simulink library "vehicle_model"  (R2018b)
settings: Solver=ode45  StartTime=0.0  StopTime=10.0  RelTol=1e-3  EnableMultiTasking=on
undefined symbols (not defined in the file): DiscIntNeverNeededParam, par_VEH, select_To_Wks_akt, stepsize, v0
libraries: $bdroot x8, pacejka_trans x6, simulink x4, body_chassis_vert x1
(part 1 of 4)
settings Model: Creator=CA-Win7Pro2  LastModifiedBy=ga35gug
settings DataIOCC: LimitDataPoints=on  SaveFormat=Array  SignalLoggingSaveFormat=ModelDataLogs
settings OptimizationCC: LifeSpan=inf
settings DebuggingCC: UnderspecifiedInitializationDetection=Classic  MergeDetectMultiDrivingBlocksExec=none  SolverPrmCheckMsg=warning  MultiTaskDSMMsg=warning  MultiTaskCondExecSysMsg=none  AllowSymbolicDim=off  SFUnexpectedBacktrackingDiag=warning  SFNoUnconditionalDefaultTransitionDiag=warning  SFExecutionAtInitializationDiag=none
settings HardwareCC: ProdBitPerPointer=32  ProdBitPerSizeT=32  ProdBitPerPtrDiffT=32  ProdLargestAtomicFloat=None  ProdIntDivRoundTo=Undefined  ProdEndianess=Unspecified  ProdWordSize=32  ProdHWDeviceType=32-bit Generic
settings ModelReferenceCC: PropagateSignalLabelsOutOfModel=off
settings SFSimCC: SimUseLocalCustomCode=off
settings RTWCC: RTWUseLocalCustomCode=off
settings CodeAppCC: StateflowObjectComments=on
settings GRTTargetCC: TargetLangStandard=C89/C90 (ANSI)  GeneratePreprocessorConditionals=Disable all
settings ConfigComp: CovMetricSettings=dw  CovHtmlReporting=on  CovSaveCumulativeToWorkspaceVar=on  CovSaveSingleToWorkspaceVar=on  CovExternalEMLEnable=off

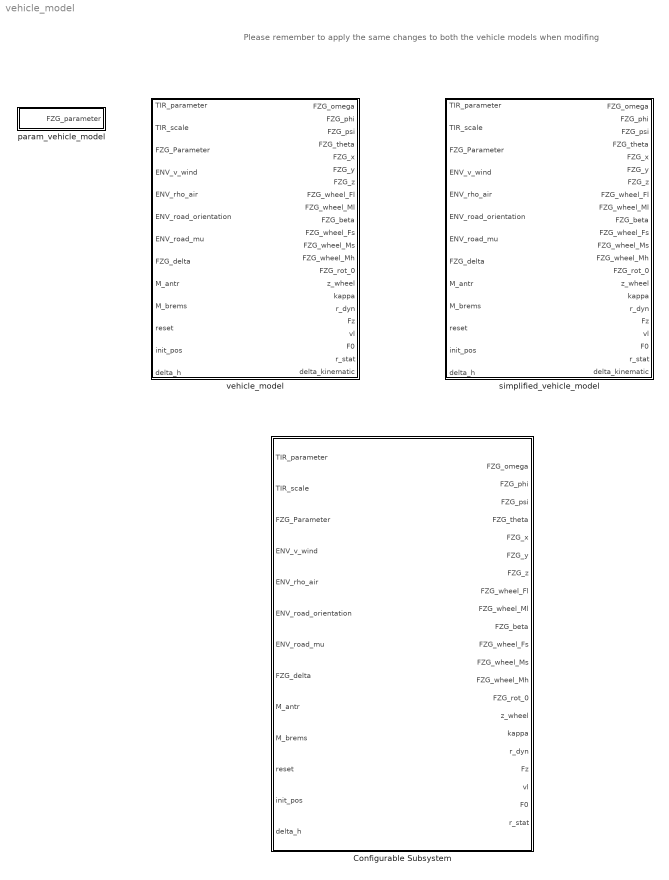
== system vehicle_model ==
  note: Please remember to apply the same changes to both the vehicle models when modifing
  Configurable Subsystem : Subsystem  BlockChoice=vehicle_model
      settings: TemplateBlock=self  MemberBlocks=simplified_vehicle_model,vehicle_model
  param_vehicle_model : Subsystem
  simplified_vehicle_model : Subsystem  TreatAsAtomicUnit=on  SystemSampleTime=stepsize
      settings: MinAlgLoopOccurrences=on
  vehicle_model : Subsystem  TreatAsAtomicUnit=on  SystemSampleTime=stepsize
      settings: MinAlgLoopOccurrences=on

== system vehicle_model/Configurable Subsystem ==
  TIR_parameter : Inport
  TIR_scale : Inport  Port=2
  FZG_Parameter : Inport  Port=3
  ENV_v_wind : Inport  Port=4
  ENV_rho_air : Inport  Port=5
  ENV_road_orientation : Inport  Port=6
  ENV_road_mu : Inport  Port=7
  FZG_delta : Inport  Port=8
  M_antr : Inport  Port=9
  M_brems : Inport  Port=10
  reset : Inport  Port=11
  init_pos : Inport  Port=12
  delta_h : Inport  Port=13
  vehicle_model : $bdroot/vehicle_model  SystemSampleTime=stepsize
  FZG_omega : Outport
  FZG_phi : Outport  Port=2
  FZG_psi : Outport  Port=3
  FZG_theta : Outport  Port=4
  FZG_x : Outport  Port=5
  FZG_y : Outport  Port=6
  FZG_z : Outport  Port=7
  FZG_wheel_Fl : Outport  Port=8
  FZG_wheel_Ml : Outport  Port=9
  FZG_beta : Outport  Port=10
  FZG_wheel_Fs : Outport  Port=11
  FZG_wheel_Ms : Outport  Port=12
  FZG_wheel_Mh : Outport  Port=13
  FZG_rot_0 : Outport  Port=14
  z_wheel : Outport  Port=15
  kappa : Outport  Port=16
  r_dyn : Outport  Port=17
  Fz : Outport  Port=18
  vl : Outport  Port=19
  F0 : Outport  Port=20
  r_stat : Outport  Port=21
  wires:
  TIR_parameter/1 -> vehicle_model/1
  TIR_scale/1 -> vehicle_model/2
  FZG_Parameter/1 -> vehicle_model/3
  ENV_v_wind/1 -> vehicle_model/4
  ENV_rho_air/1 -> vehicle_model/5
  ENV_road_orientation/1 -> vehicle_model/6
  ENV_road_mu/1 -> vehicle_model/7
  FZG_delta/1 -> vehicle_model/8
  M_antr/1 -> vehicle_model/9
  M_brems/1 -> vehicle_model/10
  reset/1 -> vehicle_model/11
  init_pos/1 -> vehicle_model/12
  delta_h/1 -> vehicle_model/13
  vehicle_model/1 -> FZG_omega/1
  vehicle_model/2 -> FZG_phi/1
  vehicle_model/3 -> FZG_psi/1
  vehicle_model/4 -> FZG_theta/1
  vehicle_model/5 -> FZG_x/1
  vehicle_model/6 -> FZG_y/1
  vehicle_model/7 -> FZG_z/1
  vehicle_model/8 -> FZG_wheel_Fl/1
  vehicle_model/9 -> FZG_wheel_Ml/1
  vehicle_model/10 -> FZG_beta/1
  vehicle_model/11 -> FZG_wheel_Fs/1
  vehicle_model/12 -> FZG_wheel_Ms/1
  vehicle_model/13 -> FZG_wheel_Mh/1
  vehicle_model/14 -> FZG_rot_0/1
  vehicle_model/15 -> z_wheel/1
  vehicle_model/16 -> kappa/1
  vehicle_model/17 -> r_dyn/1  "kappa"
  vehicle_model/18 -> Fz/1  "Fz"
  vehicle_model/19 -> vl/1  "vl"
  vehicle_model/20 -> F0/1  "F0"
  vehicle_model/21 -> r_stat/1

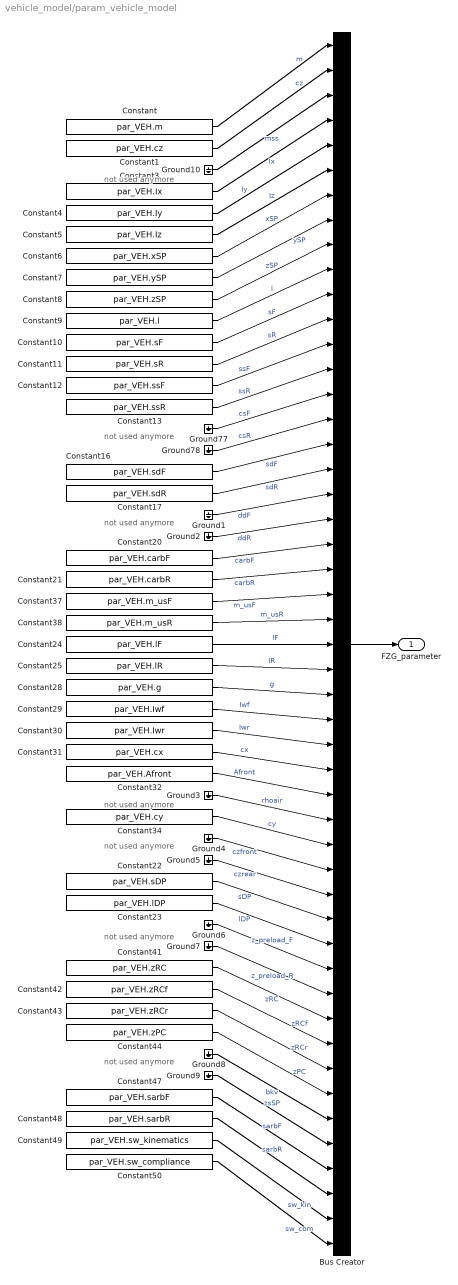
== system vehicle_model/param_vehicle_model ==
  note: not used anymore
  note: not used anymore
  note: not used anymore
  note: not used anymore
  note: not used anymore
  note: not used anymore
  note: not used anymore
  Bus Creator : BusCreator  Inputs=49
  Constant : Constant  Value=par_VEH.m
  Constant1 : Constant  Value=par_VEH.cz
  Constant10 : Constant  Value=par_VEH.sF
  Constant11 : Constant  Value=par_VEH.sR
  Constant12 : Constant  Value=par_VEH.ssF
  Constant13 : Constant  Value=par_VEH.ssR
  Constant16 : Constant  Value=par_VEH.sdF
  Constant17 : Constant  Value=par_VEH.sdR
  Constant20 : Constant  Value=par_VEH.carbF
  Constant21 : Constant  Value=par_VEH.carbR
  Constant22 : Constant  Value=par_VEH.sDP
  Constant23 : Constant  Value=par_VEH.lDP
  Constant24 : Constant  Value=par_VEH.lF
  Constant25 : Constant  Value=par_VEH.lR
  Constant28 : Constant  Value=par_VEH.g
  Constant29 : Constant  Value=par_VEH.Iwf
  Constant3 : Constant  Value=par_VEH.Ix
  Constant30 : Constant  Value=par_VEH.Iwr
  Constant31 : Constant  Value=par_VEH.cx
  Constant32 : Constant  Value=par_VEH.Afront
  Constant34 : Constant  Value=par_VEH.cy
  Constant37 : Constant  Value=par_VEH.m_usF
  Constant38 : Constant  Value=par_VEH.m_usR
  Constant4 : Constant  Value=par_VEH.Iy
  Constant41 : Constant  Value=par_VEH.zRC
  Constant42 : Constant  Value=par_VEH.zRCf
  Constant43 : Constant  Value=par_VEH.zRCr
  Constant44 : Constant  Value=par_VEH.zPC
  Constant47 : Constant  Value=par_VEH.sarbF
  Constant48 : Constant  Value=par_VEH.sarbR
  Constant49 : Constant  Value=par_VEH.sw_kinematics
  Constant5 : Constant  Value=par_VEH.Iz
  Constant50 : Constant  Value=par_VEH.sw_compliance
  Constant6 : Constant  Value=par_VEH.xSP
  Constant7 : Constant  Value=par_VEH.ySP
  Constant8 : Constant  Value=par_VEH.zSP
  Constant9 : Constant  Value=par_VEH.l
  Ground{1..10,77..78} (12 alike) : Ground
  FZG_parameter : Outport
  wires:
  Ground8/1 -> Bus Creator/44  "bkv"
  Constant30/1 -> Bus Creator/29  "Iwr"
  Constant29/1 -> Bus Creator/28  "Iwf"
  Constant28/1 -> Bus Creator/27  "g"
  Constant25/1 -> Bus Creator/26  "lR"
  Constant24/1 -> Bus Creator/25  "lF"
  Constant21/1 -> Bus Creator/22  "carbR"
  Constant20/1 -> Bus Creator/21  "carbF"
  Ground2/1 -> Bus Creator/20  "ddR"
  Ground1/1 -> Bus Creator/19  "ddF"
  Constant17/1 -> Bus Creator/18  "sdR"
  Constant16/1 -> Bus Creator/17  "sdF"
  Ground78/1 -> Bus Creator/16  "csR"
  Ground77/1 -> Bus Creator/15  "csF"
  Constant13/1 -> Bus Creator/14  "ssR"
  Constant12/1 -> Bus Creator/13  "ssF"
  Constant11/1 -> Bus Creator/12  "sR"
  Constant10/1 -> Bus Creator/11  "sF"
  Constant9/1 -> Bus Creator/10  "l"
  Constant8/1 -> Bus Creator/9  "zSP"
  Constant7/1 -> Bus Creator/8  "ySP"
  Constant6/1 -> Bus Creator/7  "xSP"
  Constant5/1 -> Bus Creator/6  "Iz"
  Constant4/1 -> Bus Creator/5  "Iy"
  Constant3/1 -> Bus Creator/4  "Ix"
  Ground10/1 -> Bus Creator/3  "mss"
  Constant/1 -> Bus Creator/1  "m"
  Bus Creator/1 -> FZG_parameter/1
  Constant31/1 -> Bus Creator/30  "cx"
  Constant32/1 -> Bus Creator/31  "Afront"
  Ground3/1 -> Bus Creator/32  "rhoair"
  Constant34/1 -> Bus Creator/33  "cy"
  Ground4/1 -> Bus Creator/34  "czfront"
  Ground5/1 -> Bus Creator/35  "czrear"
  Constant22/1 -> Bus Creator/36  "sDP"
  Constant23/1 -> Bus Creator/37  "lDP"
  Constant37/1 -> Bus Creator/23  "m_usF"
  Constant38/1 -> Bus Creator/24  "m_usR"
  Constant1/1 -> Bus Creator/2  "cz"
  Ground6/1 -> Bus Creator/38  "z_preload_F"
  Constant43/1 -> Bus Creator/42  "zRCr"
  Constant44/1 -> Bus Creator/43  "zPC"
  Constant47/1 -> Bus Creator/46  "sarbF"
  Constant48/1 -> Bus Creator/47  "sarbR"
  Constant49/1 -> Bus Creator/48  "sw_kin"
  Constant50/1 -> Bus Creator/49  "sw_com"
  Ground7/1 -> Bus Creator/39  "z_preload_R"
  Constant41/1 -> Bus Creator/40  "zRC"
  Constant42/1 -> Bus Creator/41  "zRCf"
  Ground9/1 -> Bus Creator/45  "zsSP"

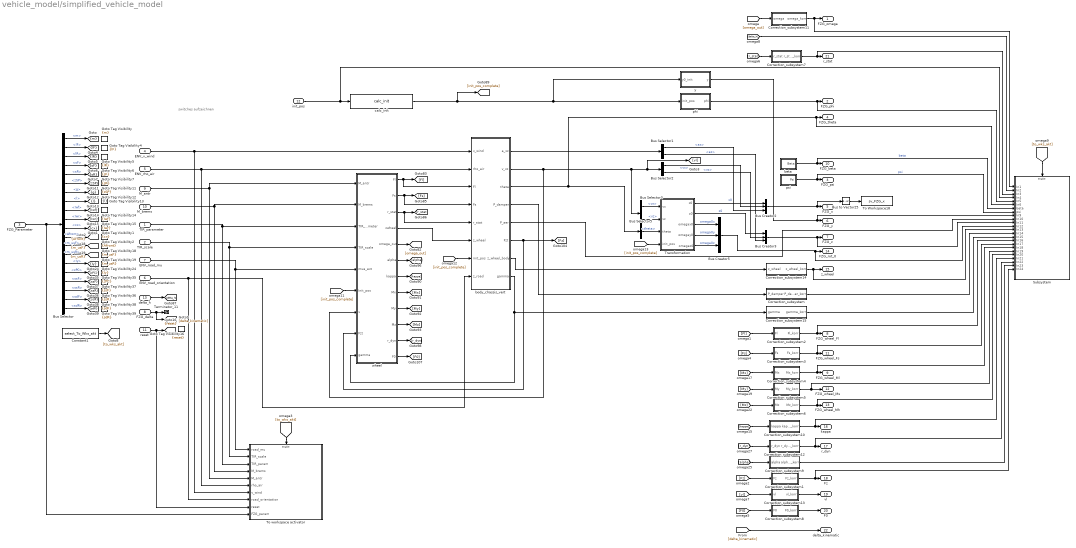
== system vehicle_model/simplified_vehicle_model ==
  note: switches aufzeichnen
  TIR_parameter : Inport
  TIR_scale : Inport  Port=2
  FZG_Parameter : Inport  Port=3
  ENV_v_wind : Inport  Port=4
  ENV_rho_air : Inport  Port=5
  ENV_road_orientation : Inport  Port=6
  ENV_road_mu : Inport  Port=7
  FZG_delta : Inport  Port=8
  M_antr : Inport  Port=9  PortDimensions=4
  M_brems : Inport  Port=10  PortDimensions=4
  reset : Inport  Port=11
  init_pos : Inport  Port=12
  delta_h : Inport  Port=13
  Bus Creator2 : BusCreator  Inputs=3
  Bus Creator3 : BusCreator  Inputs=3
  Bus Creator5 : BusCreator  Inputs=3
  Bus Selector : BusSelector  OutputSignals=m,lF,lR,sF,sR,zSP,g,l,Iwf,Iwr,cx,Afront,m_usF,m_usR,Iy,zPC,ssF,ssR,sdF,sdR
  Bus Selector1 : BusSelector  OutputSignals=ax,az
  Bus Selector2 : BusSelector  OutputSignals=vx,vz
  Bus Selector3 : BusSelector  OutputSignals=vx,vz
  Bus Selector5 : BusSelector  OutputSignals=theta
  Bus to Vector25 : BusToVector
  Constant1 : Constant  Value=select_To_Wks_akt
  Correction_subsystem : Subsystem
  Correction_subsystem1 : Subsystem
  Correction_subsystem10 : Subsystem
  Correction_subsystem11 : Subsystem
  Correction_subsystem12 : Subsystem
  Correction_subsystem13 : Subsystem
  Correction_subsystem14 : Subsystem
  Correction_subsystem15 : Subsystem
  Correction_subsystem2 : Subsystem
  Correction_subsystem3 : Subsystem
  Correction_subsystem4 : Subsystem
  Correction_subsystem5 : Subsystem
  Correction_subsystem6 : Subsystem
  Correction_subsystem7 : Subsystem
  Correction_subsystem8 : Subsystem
  Correction_subsystem9 : Subsystem
  Goto Tag Visibility : GotoTagVisibility  GotoTag=m
  Goto Tag Visibility1 : GotoTagVisibility  GotoTag=cx
  Goto Tag Visibility11 : GotoTagVisibility  GotoTag=zSP
  Goto Tag Visibility12 : GotoTagVisibility  GotoTag=g
  Goto Tag Visibility13 : GotoTagVisibility  GotoTag=l
  Goto Tag Visibility14 : GotoTagVisibility  GotoTag=Iwf
  Goto Tag Visibility15 : GotoTagVisibility  GotoTag=Iwr
  Goto Tag Visibility16 : GotoTagVisibility  GotoTag=reset
  Goto Tag Visibility18 : GotoTagVisibility  GotoTag=m_usF
  Goto Tag Visibility19 : GotoTagVisibility  GotoTag=m_usR
  Goto Tag Visibility2 : GotoTagVisibility  GotoTag=Afront
  Goto Tag Visibility24 : GotoTagVisibility  GotoTag=Iy
  Goto Tag Visibility35 : GotoTagVisibility  GotoTag=zPC
  Goto Tag Visibility36 : GotoTagVisibility  GotoTag=ssR
  Goto Tag Visibility37 : GotoTagVisibility  GotoTag=ssF
  Goto Tag Visibility38 : GotoTagVisibility  GotoTag=sdF
  Goto Tag Visibility39 : GotoTagVisibility  GotoTag=sdR
  Goto Tag Visibility4 : GotoTagVisibility  GotoTag=lF
  Goto Tag Visibility5 : GotoTagVisibility  GotoTag=lR
  Goto Tag Visibility6 : GotoTagVisibility  GotoTag=sF
  Goto Tag Visibility7 : GotoTagVisibility  GotoTag=sR
  Subsystem : Subsystem
  Terminator_11 : Terminator
  To Workspace18 : ToWorkspace  VariableName=sv_FZG_x  SampleTime=-1
      settings: Decimation=savedec  Save2DSignal=2-D array (concatenate along first dimension)
  To workspace activator : Subsystem
  Transformation : Subsystem
  beta : Subsystem
  body_chassis_vert : Subsystem
  calc_init : $bdroot/vehicle_model/calc_init  SystemSampleTime=-1
  "phi " : Subsystem
  psi : Subsystem
  wheel : Subsystem
  y : Subsystem
  FZG_omega : Outport
  FZG_phi : Outport  Port=2
  FZG_psi : Outport  Port=3
  FZG_theta : Outport  Port=4
  FZG_x : Outport  Port=5  PortDimensions=3
  FZG_y : Outport  Port=6
  FZG_z : Outport  Port=7
  FZG_wheel_Fl : Outport  Port=8
  FZG_wheel_Ml : Outport  Port=9
  FZG_beta : Outport  Port=10
  FZG_wheel_Fs : Outport  Port=11
  FZG_wheel_Ms : Outport  Port=12
  FZG_wheel_Mh : Outport  Port=13
  FZG_rot_0 : Outport  Port=14
  z_wheel : Outport  Port=15
  kappa : Outport  Port=16
  r_dyn : Outport  Port=17
  Fz : Outport  Port=18
  vl : Outport  Port=19
  F0 : Outport  Port=20
  r_stat : Outport  Port=21
  delta_kinematic : Outport  Port=22
  tag scope: Afront=scoped, Iwf=scoped, Iwr=scoped, Iy=scoped, cx=scoped, g=scoped, l=scoped, lF=scoped, lR=scoped, m=scoped, m_usF=scoped, m_usR=scoped, reset=scoped, sF=scoped, sR=scoped, sdF=scoped, sdR=scoped, ssF=scoped, ssR=scoped, zPC=scoped, zSP=scoped
  wires:
  Transformation/5(omegaz0) -> Bus Creator5/3  "omega0z"
  Bus Selector1/2 -> Bus Creator3/3  "<az>"
  Correction_subsystem7/1(r_stat_korr) -> Subsystem/3(In3), r_stat/1
  Correction_subsystem1/1(Fz_korr) -> Subsystem/24(In24), Fz/1
  body_chassis_vert/1(a_xz) -> Bus Selector1/1
  Correction_subsystem13/1(vl_korr) -> vl/1
  [vl] -> Correction_subsystem13/1(vl)
  Bus Selector3/2 -> Transformation/2(vz)  "<vz>"
  [init_pos_complete] -> Transformation/4(init_pos)
  Transformation/1(x0) -> Bus Creator2/1  "x0"
  Correction_subsystem12/1(r_dyn_korr) -> Subsystem/22(In22), r_dyn/1
  Bus Selector3/1 -> Transformation/1(vx)  "<vx>"
  Transformation/3(omegax0) -> Bus Creator5/1  "omega0x"
  Bus Selector5/1 -> Transformation/3(theta)  "<theta>"
  body_chassis_vert/7(z_wheel_body) -> Correction_subsystem14/1(z_wheel)
  Correction_subsystem3/1(Fs_korr) -> Subsystem/17(In17), FZG_wheel_Fs/1
  Correction_subsystem2/1(Fl_korr) -> Subsystem/16(In16), FZG_wheel_Fl/1
  Bus Selector/13 -> [m_usF]  "<m_usF>"
  body_chassis_vert/4(P_damper) -> Correction_subsystem/1(P_damper)
  wheel/5(omega_out) -> [omega_out]
  Bus Selector2/1 -> Bus Creator2/2  "<vx>"
  wheel/4(zwheel) -> body_chassis_vert/6(z_wheel)
  TIR_parameter/1 -> wheel/3(TIR_parameter), To workspace activator/3(TIR_param)
  Bus Selector/19 -> [sdF]  "<sdF>"
  Bus Selector/7 -> [g]  "<g>"
  [init_pos_complete] -> wheel/6(Init_pos)
  Bus Selector/15 -> [Iy]  "<Iy>"
  Correction_subsystem11/1(omega_korr) -> Subsystem/1(In1), FZG_omega/1
  Transformation/4(omegay0) -> Bus Creator5/2  "omega0y"
  ENV_road_mu/1 -> wheel/5(mue_ext), To workspace activator/1(road_mu)
  body_chassis_vert/6(Fzt) -> wheel/8(Fzt), [Fz]
  Bus Selector/14 -> [m_usR]  "<m_usR>"
  calc_init/1 -> [init_pos_complete], y/1(y0_init), "phi "/1(init_pos)
  delta_h/1 -> [delta_h]
  Bus Selector/4 -> [sF]  "<sF>"
  Bus Selector1/1 -> Bus Creator2/3  "<ax>"
  M_brems/1 -> To workspace activator/4(M_brems), wheel/2(M_brems)
  reset/1 -> To workspace activator/9(reset), [reset]
  body_chassis_vert/2(v_xz) -> wheel/7(v), Bus Selector3/1, [vl], Bus Selector2/1
  M_antr/1 -> To workspace activator/5(M_antr), wheel/1(M_antr)
  [omega_out] -> Correction_subsystem11/1(omega)
  Bus Selector/8 -> [l]  "<l>"
  TIR_scale/1 -> wheel/4(TIR_scale), To workspace activator/2(TIR_scale)
  ENV_rho_air/1 -> To workspace activator/6(rho_air), body_chassis_vert/2(rho_air)
  wheel/1(Fl) -> body_chassis_vert/3(Fl), [Fl]
  Bus Selector/10 -> [Iwr]  "<Iwr>"
  Bus Selector/2 -> [lF]  "<lF>"
  Bus Selector/18 -> [ssR]  "<ssR>"
  Bus Selector/3 -> [lR]  "<lR>"
  Bus Selector/1 -> [m]  "<m>"
  ENV_v_wind/1 -> To workspace activator/7(v_wind), body_chassis_vert/1(v_wind)
  init_pos/1 -> Subsystem/4(In4), calc_init/1
  wheel/10(Mz) -> [Mz]
  [r_stat] -> Correction_subsystem7/1(r_stat)
  Bus Selector/20 -> [sdR]  "<sdR>"
  Bus Selector/17 -> [ssF]  "<ssF>"
  [Mx] -> Correction_subsystem4/1(Mx)
  [kappa] -> Correction_subsystem10/1(kappa)
  [Mz] -> Correction_subsystem6/1(Mz)
  [F0] -> Correction_subsystem8/1(F0)
  Bus to Vector25/1 -> To Workspace18/1
  Bus Selector/12 -> [Afront]  "<Afront>"
  [My] -> Correction_subsystem5/1(My)
  wheel/12(F0) -> [F0]
  [r_dyn] -> Correction_subsystem12/1(r_dyn)
  Bus Selector/16 -> [zPC]  "<zPC>"
  [init_pos_complete] -> body_chassis_vert/7(init_pos)
  wheel/3(r_stat) -> body_chassis_vert/5(r_stat), [r_stat]
  wheel/8(Mx) -> [Mx]
  wheel/9(My) -> [My]
  body_chassis_vert/8(gamma) -> wheel/9(gamma), Correction_subsystem15/1(gamma)
  wheel/7(kappa) -> [kappa]
  Bus Creator2/1 -> FZG_x/1, Bus to Vector25/1
  wheel/11(r_dyn) -> [r_dyn]
  Transformation/2(z0) -> Bus Creator3/1  "z0"
  Bus Selector/11 -> [cx]  "<cx>"
  Correction_subsystem6/1(Mz_korr) -> Subsystem/20(In20), FZG_wheel_Mh/1
  body_chassis_vert/3(theta) -> Bus Selector5/1, Subsystem/6(In6), FZG_theta/1
  Correction_subsystem4/1(Mx_korr) -> Subsystem/18(In18), FZG_wheel_Ml/1
  ENV_road_orientation/1 -> To workspace activator/8(road_orientation), body_chassis_vert/8(z_road)
  Bus Creator3/1 -> Subsystem/11(In11), FZG_z/1
  Bus Creator5/1 -> Subsystem/12(In12), FZG_rot_0/1
  "phi "/1(phi) -> Subsystem/5(In5), FZG_phi/1
  Correction_subsystem5/1(My_korr) -> Subsystem/19(In19), FZG_wheel_Ms/1
  Bus Selector2/2 -> Bus Creator3/2  "<vz>"
  FZG_Parameter/1 -> To workspace activator/10(FZG_param), Bus Selector/1
  Bus Selector/9 -> [Iwf]  "<Iwf>"
  Correction_subsystem10/1(kappa_korr) -> Subsystem/21(In21), kappa/1
  FZG_delta/1 -> [delta_kinematic], Terminator_11/1
  Bus Selector/6 -> [zSP]  "<zSP>"
  Bus Selector/5 -> [sR]  "<sR>"
  [Fl] -> Correction_subsystem2/1(Fl)
  Correction_subsystem8/1(F0_korr) -> F0/1
  Correction_subsystem14/1(z_wheel_korr) -> Subsystem/13(In13), z_wheel/1
  [Fz] -> Correction_subsystem1/1(Fz)
  [Fs] -> Correction_subsystem3/1(Fs)
  wheel/2(Fs) -> body_chassis_vert/4(Fs), [Fs]
  beta/1(Beta) -> Subsystem/7(beta), FZG_beta/1  "beta"
  psi/1(Psi) -> Subsystem/8(psi), FZG_psi/1  "psi"
  y/1(y) -> Subsystem/9(In9), FZG_y/1
  [alpha] -> Correction_subsystem9/1(alpha)
  wheel/6(alpha) -> [alpha]
  [delta_h] -> Subsystem/2(In2)
  body_chassis_vert/5(P_aer) -> Subsystem/10(In10)
  Correction_subsystem/1(P_damper_korr) -> Subsystem/14(In14)
  Correction_subsystem15/1(gamma_korr) -> Subsystem/15(In15)
  Correction_subsystem9/1(alpha_korr) -> Subsystem/23(In23)
  [to_wks_akt] -> To workspace activator/Enable
  [to_wks_akt] -> Subsystem/Enable
  Constant1/1 -> [to_wks_akt]
  [delta_kinematic] -> delta_kinematic/1

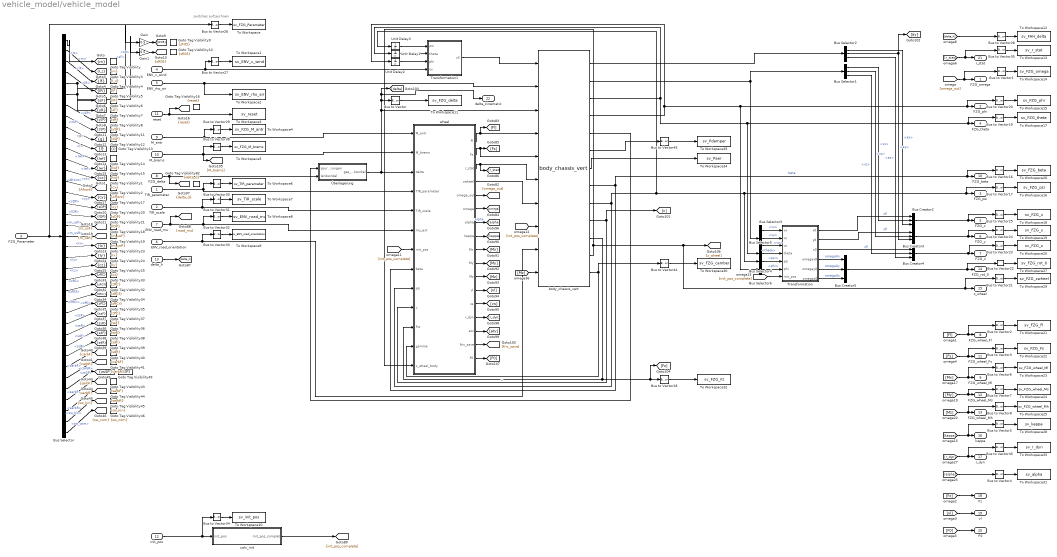
== system vehicle_model/vehicle_model ==
  note: switches aufzeichnen
  TIR_parameter : Inport
  TIR_scale : Inport  Port=2
  FZG_Parameter : Inport  Port=3
  ENV_v_wind : Inport  Port=4
  ENV_rho_air : Inport  Port=5
  ENV_road_orientation : Inport  Port=6
  ENV_road_mu : Inport  Port=7
  FZG_delta : Inport  Port=8
  M_antr : Inport  Port=9  PortDimensions=4
  M_brems : Inport  Port=10  PortDimensions=4
  reset : Inport  Port=11
  init_pos : Inport  Port=12
  delta_h : Inport  Port=13
  Bus Creator{2..5} (4 alike) : BusCreator  Inputs=3
  Bus Selector : BusSelector  OutputSignals=m,Iz,lF,lR,sF,sR,ySP,zSP,g,l,Iwf,Iwr,cx,Afront,cy,sDP,lDP,m_usF,m_usR,Ix,Iy,cz,zRC,zRCf,zRCr,zPC,ssF,ssR,sdF,sdR,carbF,carbR,zsSP,sarbF,sarbR,sw_kin,sw_com
  Bus Selector1 : BusSelector  OutputSignals=vx,vy,vz
  Bus Selector2 : BusSelector  OutputSignals=ax,ay,az
  Bus Selector3 : BusSelector  OutputSignals=vx,vy,vz
  Bus Selector4 : BusSelector  OutputSignals=psi
  Bus Selector5 : BusSelector  OutputSignals=theta
  Bus Selector6 : BusSelector  OutputSignals=phi
  Bus to Vector{,1..8,16..35,38,43..45} (33 alike) : BusToVector
  Gain : Gain  Gain=0.5
  Gain1 : Gain  Gain=0.5
  Goto Tag Visibility : GotoTagVisibility  GotoTag=m
  Goto Tag Visibility1 : GotoTagVisibility  GotoTag=cx
  Goto Tag Visibility10 : GotoTagVisibility  GotoTag=sR05
  Goto Tag Visibility11 : GotoTagVisibility  GotoTag=zSP
  Goto Tag Visibility12 : GotoTagVisibility  GotoTag=g
  Goto Tag Visibility13 : GotoTagVisibility  GotoTag=l
  Goto Tag Visibility14 : GotoTagVisibility  GotoTag=Iwf
  Goto Tag Visibility15 : GotoTagVisibility  GotoTag=Iwr
  Goto Tag Visibility16 : GotoTagVisibility  GotoTag=reset
  Goto Tag Visibility17 : GotoTagVisibility  GotoTag=cy
  Goto Tag Visibility18 : GotoTagVisibility  GotoTag=m_usF
  Goto Tag Visibility19 : GotoTagVisibility  GotoTag=m_usR
  Goto Tag Visibility2 : GotoTagVisibility  GotoTag=Afront
  Goto Tag Visibility20 : GotoTagVisibility  GotoTag=sDP
  Goto Tag Visibility21 : GotoTagVisibility  GotoTag=lDP
  Goto Tag Visibility23 : GotoTagVisibility  GotoTag=Ix
  Goto Tag Visibility24 : GotoTagVisibility  GotoTag=Iy
  Goto Tag Visibility25 : GotoTagVisibility  GotoTag=cz
  Goto Tag Visibility3 : GotoTagVisibility  GotoTag=I_z
  Goto Tag Visibility32 : GotoTagVisibility  GotoTag=zRCf
  Goto Tag Visibility33 : GotoTagVisibility  GotoTag=zRC
  Goto Tag Visibility34 : GotoTagVisibility  GotoTag=zRCr
  Goto Tag Visibility35 : GotoTagVisibility  GotoTag=zPC
  Goto Tag Visibility36 : GotoTagVisibility  GotoTag=ssR
  Goto Tag Visibility37 : GotoTagVisibility  GotoTag=ssF
  Goto Tag Visibility38 : GotoTagVisibility  GotoTag=sdF
  Goto Tag Visibility39 : GotoTagVisibility  GotoTag=sdR
  Goto Tag Visibility4 : GotoTagVisibility  GotoTag=lF
  Goto Tag Visibility40 : GotoTagVisibility  GotoTag=carbF
  Goto Tag Visibility41 : GotoTagVisibility  GotoTag=carbR
  Goto Tag Visibility43 : GotoTagVisibility  GotoTag=sarbF
  Goto Tag Visibility44 : GotoTagVisibility  GotoTag=sarbR
  Goto Tag Visibility45 : GotoTagVisibility  GotoTag=sw_kin
  Goto Tag Visibility46 : GotoTagVisibility  GotoTag=sw_com
  Goto Tag Visibility49 : GotoTagVisibility  GotoTag=zsSP
  Goto Tag Visibility5 : GotoTagVisibility  GotoTag=lR
  Goto Tag Visibility6 : GotoTagVisibility  GotoTag=sF
  Goto Tag Visibility7 : GotoTagVisibility  GotoTag=sR
  Goto Tag Visibility8 : GotoTagVisibility  GotoTag=ySP
  Goto Tag Visibility82 : GotoTagVisibility  GotoTag=delta_d
  Goto Tag Visibility9 : GotoTagVisibility  GotoTag=sF05
  To Workspace : ToWorkspace  VariableName=sv_FZG_Parameter  SampleTime=-1
      settings: MaxDataPoints=1  Decimation=savedec  Save2DSignal=2-D array (concatenate along first dimension)
  To Workspace1 : ToWorkspace  VariableName=sv_ENV_v_wind  SampleTime=-1
      settings: Decimation=savedec  Save2DSignal=2-D array (concatenate along first dimension)
  To Workspace10 : ToWorkspace  VariableName=sv_init_pos  SampleTime=-1
      settings: MaxDataPoints=1  Decimation=savedec  Save2DSignal=2-D array (concatenate along first dimension)
  To Workspace11 : ToWorkspace  VariableName=sv_FZG_delta  SampleTime=-1
      settings: Decimation=savedec  Save2DSignal=2-D array (concatenate along first dimension)
  To Workspace12 : ToWorkspace  VariableName=sv_FAH_delta  SampleTime=-1
      settings: Decimation=savedec  Save2DSignal=2-D array (concatenate along first dimension)
  To Workspace13 : ToWorkspace  VariableName=sv_r_stat  SampleTime=-1
      settings: Decimation=savedec  Save2DSignal=2-D array (concatenate along first dimension)
  To Workspace14 : ToWorkspace  VariableName=sv_FZG_omega  SampleTime=-1
      settings: Decimation=savedec  Save2DSignal=2-D array (concatenate along first dimension)
  To Workspace15 : ToWorkspace  VariableName=sv_FZG_phi  SampleTime=-1
      settings: Decimation=savedec  Save2DSignal=2-D array (concatenate along first dimension)
  To Workspace16 : ToWorkspace  VariableName=sv_FZG_psi  SampleTime=-1
      settings: Decimation=savedec  Save2DSignal=2-D array (concatenate along first dimension)
  To Workspace17 : ToWorkspace  VariableName=sv_FZG_theta  SampleTime=-1
      settings: Decimation=savedec  Save2DSignal=2-D array (concatenate along first dimension)
  To Workspace18 : ToWorkspace  VariableName=sv_FZG_x  SampleTime=-1
      settings: Decimation=savedec  Save2DSignal=2-D array (concatenate along first dimension)
  To Workspace19 : ToWorkspace  VariableName=sv_FZG_y  SampleTime=-1
      settings: Decimation=savedec  Save2DSignal=2-D array (concatenate along first dimension)
  To Workspace2 : ToWorkspace  VariableName=sv_ENV_rho_air  SampleTime=-1
      settings: Decimation=savedec  Save2DSignal=2-D array (concatenate along first dimension)
  To Workspace20 : ToWorkspace  VariableName=sv_FZG_z  SampleTime=-1
      settings: Decimation=savedec  Save2DSignal=2-D array (concatenate along first dimension)
  To Workspace21 : ToWorkspace  VariableName=sv_FZG_Fl  SampleTime=-1
      settings: Decimation=savedec  Save2DSignal=2-D array (concatenate along first dimension)
  To Workspace22 : ToWorkspace  VariableName=sv_FZG_Fs  SampleTime=-1
      settings: Decimation=savedec  Save2DSignal=2-D array (concatenate along first dimension)
  To Workspace23 : ToWorkspace  VariableName=sv_FZG_wheel_Ml  SampleTime=-1
      settings: Decimation=savedec  Save2DSignal=2-D array (concatenate along first dimension)
  To Workspace24 : ToWorkspace  VariableName=sv_FZG_wheel_Ms  SampleTime=-1
      settings: Decimation=savedec  Save2DSignal=2-D array (concatenate along first dimension)
  To Workspace25 : ToWorkspace  VariableName=sv_FZG_wheel_Mh  SampleTime=-1
      settings: Decimation=savedec  Save2DSignal=2-D array (concatenate along first dimension)
  To Workspace26 : ToWorkspace  VariableName=sv_FZG_beta  SampleTime=-1
      settings: Decimation=savedec  Save2DSignal=2-D array (concatenate along first dimension)
  To Workspace27 : ToWorkspace  VariableName=sv_FZG_rot_0  SampleTime=-1
      settings: Decimation=savedec  Save2DSignal=2-D array (concatenate along first dimension)
  To Workspace28 : ToWorkspace  VariableName=sv_kappa  SampleTime=-1
      settings: Decimation=savedec  Save2DSignal=2-D array (concatenate along first dimension)
  To Workspace29 : ToWorkspace  VariableName=sv_FZG_zwheel  SampleTime=-1
      settings: Decimation=savedec  Save2DSignal=2-D array (concatenate along first dimension)
  To Workspace3 : ToWorkspace  VariableName=sv_reset  SampleTime=-1
      settings: Decimation=savedec  Save2DSignal=2-D array (concatenate along first dimension)
  To Workspace30 : ToWorkspace  VariableName=sv_FZG_camber  SampleTime=-1
      settings: Decimation=savedec  Save2DSignal=2-D array (concatenate along first dimension)
  To Workspace31 : ToWorkspace  VariableName=sv_alpha  SampleTime=-1
      settings: Decimation=savedec  Save2DSignal=2-D array (concatenate along first dimension)
  To Workspace32 : ToWorkspace  VariableName=sv_FZG_Fz  SampleTime=-1
      settings: Decimation=savedec  Save2DSignal=2-D array (concatenate along first dimension)
  To Workspace33 : ToWorkspace  VariableName=sv_r_dyn  SampleTime=-1
      settings: Decimation=savedec  Save2DSignal=2-D array (concatenate along first dimension)
  To Workspace34 : ToWorkspace  VariableName=sv_Paer  SampleTime=-1
      settings: Decimation=savedec  Save2DSignal=2-D array (concatenate along first dimension)
  To Workspace35 : ToWorkspace  VariableName=sv_Pdamper  SampleTime=-1
      settings: Decimation=savedec  Save2DSignal=2-D array (concatenate along first dimension)
  To Workspace4 : ToWorkspace  VariableName=sv_FZG_M_antr  SampleTime=-1
      settings: Decimation=savedec  Save2DSignal=2-D array (concatenate along first dimension)
  To Workspace5 : ToWorkspace  VariableName=sv_FZG_M_brems  SampleTime=-1
      settings: Decimation=savedec  Save2DSignal=2-D array (concatenate along first dimension)
  To Workspace6 : ToWorkspace  VariableName=sv_TIR_parameter  SampleTime=-1
      settings: MaxDataPoints=1  Decimation=savedec  Save2DSignal=2-D array (concatenate along first dimension)
  To Workspace7 : ToWorkspace  VariableName=sv_TIR_scale  SampleTime=-1
      settings: MaxDataPoints=1  Decimation=savedec  Save2DSignal=2-D array (concatenate along first dimension)
  To Workspace8 : ToWorkspace  VariableName=sv_ENV_road_mu  SampleTime=-1
      settings: Decimation=savedec  Save2DSignal=2-D array (concatenate along first dimension)
  To Workspace9 : ToWorkspace  VariableName=sv_ENV_road_orientation  SampleTime=-1
      settings: Decimation=savedec  Save2DSignal=2-D array (concatenate along first dimension)
  Transformation : Subsystem
  Transformation1 : Subsystem
  Unit Delay1 : UnitDelay  SampleTime=-1
  Unit Delay2 : UnitDelay  SampleTime=-1
  Unit Delay3 : UnitDelay  SampleTime=-1
  body_chassis_vert : body_chassis_vert/body_chassis_vert  SystemSampleTime=-1
  calc_init : Subsystem
  wheel : Subsystem
  Überlagerung : Subsystem
  FZG_omega : Outport
  FZG_phi : Outport  Port=2
  FZG_psi : Outport  Port=3
  FZG_theta : Outport  Port=4
  FZG_x : Outport  Port=5  PortDimensions=3
  FZG_y : Outport  Port=6
  FZG_z : Outport  Port=7
  FZG_wheel_Fl : Outport  Port=8
  FZG_wheel_Ml : Outport  Port=9
  FZG_beta : Outport  Port=10
  FZG_wheel_Fs : Outport  Port=11
  FZG_wheel_Ms : Outport  Port=12
  FZG_wheel_Mh : Outport  Port=13
  FZG_rot_0 : Outport  Port=14
  z_wheel : Outport  Port=15
  kappa : Outport  Port=16
  r_dyn : Outport  Port=17
  Fz : Outport  Port=18
  vl : Outport  Port=19
  F0 : Outport  Port=20
  r_stat : Outport  Port=21
  delta_kinematic : Outport  Port=22
  tag scope: Afront=scoped, I_z=scoped, Iwf=scoped, Iwr=scoped, Ix=scoped, Iy=scoped, carbF=scoped, carbR=scoped, cx=scoped, cy=scoped, cz=scoped, delta_d=scoped, g=scoped, l=scoped, lDP=scoped, lF=scoped, lR=scoped, m=scoped, m_usF=scoped, m_usR=scoped, reset=scoped, sDP=scoped, sF05=scoped, sF=scoped, sR05=scoped, sR=scoped, sarbF=scoped, sarbR=scoped, sdF=scoped, sdR=scoped, ssF=scoped, ssR=scoped, sw_com=scoped, sw_kin=scoped, ySP=scoped, zPC=scoped, zRC=scoped, zRCf=scoped, zRCr=scoped, zSP=scoped, zsSP=scoped
  wires:
  Gain1/1 -> [sR05]
  Gain/1 -> [sF05]
  wheel/17(F0) -> [F0]
  [vl] -> vl/1
  [Fz] -> Fz/1
  [Mz] -> body_chassis_vert/10
  delta_h/1 -> [delta_h]
  body_chassis_vert/5 -> Überlagerung/1(spuraenderungen)
  body_chassis_vert/13 -> wheel/12(gamma), Bus to Vector44/1
  wheel/15(atv) -> [atv]
  [r_dyn] -> Bus to Vector45/1, r_dyn/1
  wheel/14(r_dyn) -> [r_dyn]
  [alpha] -> Bus to Vector4/1
  wheel/7(alpha) -> [alpha]  "alpha"
  wheel/13(vs) -> [vs]
  wheel/12(vl) -> [vl]
  [Mz] -> FZG_wheel_Mh/1, Bus to Vector8/1
  wheel/11(Mz) -> [Mz]
  [My] -> FZG_wheel_Ms/1, Bus to Vector7/1
  wheel/10(My) -> [My]
  [Mx] -> FZG_wheel_Ml/1, Bus to Vector6/1
  wheel/9(Mx) -> [Mx]
  wheel/3(r_stat) -> [r_stat], body_chassis_vert/6
  [kappa] -> Bus to Vector5/1, kappa/1
  Bus to Vector5/1 -> To Workspace28/1
  wheel/8(kappa) -> [kappa]
  [init_pos_complete] -> Transformation/7(init_pos)
  [init_pos_complete] -> body_chassis_vert/8
  [init_pos_complete] -> wheel/7(init_pos)
  calc_init/1(init_pos_complete) -> [init_pos_complete]
  TIR_parameter/1 -> wheel/4(TIR_parameter), Bus to Vector30/1
  [delta_h] -> Bus to Vector28/1
  Bus to Vector28/1 -> To Workspace12/1
  [r_stat] -> r_stat/1, Bus to Vector35/1
  [Fs] -> FZG_wheel_Fs/1, Bus to Vector3/1
  wheel/6(omega) -> [omega]
  [Fl] -> FZG_wheel_Fl/1, Bus to Vector2/1
  [omega_out] -> FZG_omega/1, Bus to Vector1/1
  wheel/5(omega_out) -> [omega_out]
  body_chassis_vert/7 -> To Workspace34/1
  Bus to Vector45/1 -> To Workspace33/1
  Bus to Vector44/1 -> To Workspace30/1
  Bus to Vector43/1 -> To Workspace35/1
  body_chassis_vert/6 -> Bus to Vector43/1
  Bus Selector/13 -> [cx]  "<cx>"
  Bus Selector/14 -> [Afront]  "<Afront>"
  Bus Selector/17 -> [lDP]  "<lDP>"
  Bus Selector/18 -> [m_usF]  "<m_usF>"
  Bus Selector/26 -> [zPC]  "<zPC>"
  M_antr/1 -> Bus to Vector29/1, wheel/1(M_antr)
  M_brems/1 -> [M_brems], wheel/2(M_brems), Bus to Vector38/1
  Bus to Vector38/1 -> To Workspace5/1
  Bus Selector/33 -> [zsSP]  "<zsSP>"
  Bus to Vector35/1 -> To Workspace13/1
  Bus to Vector34/1 -> To Workspace10/1
  Bus to Vector33/1 -> To Workspace9/1
  Bus to Vector32/1 -> To Workspace8/1
  Bus to Vector31/1 -> To Workspace7/1
  Bus to Vector30/1 -> To Workspace6/1
  Bus to Vector29/1 -> To Workspace4/1
  Bus to Vector27/1 -> To Workspace1/1
  Bus to Vector26/1 -> To Workspace/1
  Bus Selector/37 -> [sw_com]  "<sw_com>"
  Bus Selector/36 -> [sw_kin]  "<sw_kin>"
  Bus Selector/34 -> [sarbF]  "<sarbF>"
  body_chassis_vert/12 -> wheel/13(z_wheel_body), [z_wheel], Bus to Vector21/1, z_wheel/1
  Bus Selector/32 -> [carbR]  "<carbR>"
  Bus Selector/31 -> [carbF]  "<carbF>"
  Bus Selector/30 -> [sdR]  "<sdR>"
  Bus Selector/29 -> [sdF]  "<sdF>"
  Bus Selector/28 -> [ssR]  "<ssR>"
  Bus Selector/27 -> [ssF]  "<ssF>"
  Bus Selector/25 -> [zRCr]  "<zRCr>"
  Bus Selector/24 -> [zRCf]  "<zRCf>"
  Bus Selector/23 -> [zRC]  "<zRC>"
  Bus Selector6/1 -> Transformation/6(phi)  "<phi>"
  Bus Selector5/1 -> Transformation/4(theta)  "<theta>"
  body_chassis_vert/4 -> Bus to Vector20/1, FZG_phi/1, Bus Selector6/1, Unit Delay2/1
  body_chassis_vert/3 -> Bus Selector5/1, Bus to Vector19/1, FZG_theta/1, Unit Delay1/1
  Bus Selector/22 -> [cz]  "<cz>"
  Bus Selector/21 -> [Iy]  "<Iy>"
  Bus Selector/20 -> [Ix]  "<Ix>"
  body_chassis_vert/1 -> Bus Selector2/1
  body_chassis_vert/2 -> Bus Selector3/1, Bus Selector1/1
  wheel/4(zwheel) -> body_chassis_vert/7
  Bus Selector/19 -> [m_usR]  "<m_usR>"
  Bus Selector/16 -> [sDP]  "<sDP>"
  Bus Selector/15 -> [cy]  "<cy>"
  Unit Delay2/1 -> Transformation1/3(phi)
  Unit Delay1/1 -> Transformation1/2(theta)
  Unit Delay3/1 -> Transformation1/1(psi)
  Transformation1/1(x3) -> body_chassis_vert/1
  init_pos/1 -> Bus to Vector34/1, calc_init/1(init_pos)
  Bus Creator5/1 -> FZG_rot_0/1, Bus to Vector22/1
  Transformation/6(omegaz0) -> Bus Creator5/3  "omega0z"
  Transformation/5(omegay0) -> Bus Creator5/2  "omega0y"
  Transformation/4(omegax0) -> Bus Creator5/1  "omega0x"
  ENV_road_mu/1 -> wheel/6(mu_ext), Bus to Vector32/1, [road_mu]
  TIR_scale/1 -> Bus to Vector31/1, wheel/5(TIR_scale)
  Bus Selector4/1 -> Transformation/5(psi)  "<psi>"
  Bus Selector3/3 -> Transformation/3(vz)  "<vz>"
  Bus Selector3/2 -> Transformation/2(vy)  "<vy>"
  Bus Selector3/1 -> Transformation/1(vx)  "<vx>"
  Transformation/3(z0) -> Bus Creator4/1  "z0"
  Transformation/2(y0) -> Bus Creator3/1  "y0"
  Transformation/1(x0) -> Bus Creator2/1  "x0"
  ENV_road_orientation/1 -> body_chassis_vert/9, Bus to Vector33/1
  ENV_rho_air/1 -> To Workspace2/1, body_chassis_vert/2
  ENV_v_wind/1 -> Bus to Vector27/1, Transformation1/4(vx)
  FZG_Parameter/1 -> Bus Selector/1, Bus to Vector26/1
  wheel/2(Fs) -> [Fs], body_chassis_vert/5
  body_chassis_vert/8 -> wheel/8(beta), FZG_beta/1, Bus to Vector16/1  "beta"
  body_chassis_vert/10 -> wheel/10(v), [v]  "v"
  Bus Selector/1 -> [m]  "<m>"
  Bus Creator4/1 -> Bus to Vector23/1, FZG_z/1
  Bus Creator3/1 -> Bus to Vector24/1, FZG_y/1
  Bus Creator2/1 -> Bus to Vector25/1, FZG_x/1
  Bus Selector/2 -> [I_z]  "<Iz>"
  Bus Selector/3 -> [lF]  "<lF>"
  Bus Selector/4 -> [lR]  "<lR>"
  Bus Selector/5 -> [sF], Gain/1  "<sF>"
  Bus Selector/6 -> [sR], Gain1/1  "<sR>"
  Bus Selector/7 -> [ySP]  "<ySP>"
  body_chassis_vert/9 -> wheel/9(psi), Bus to Vector17/1, FZG_psi/1, Bus Selector4/1, Unit Delay3/1
  Bus Selector/8 -> [zSP]  "<zSP>"
  Bus Selector/9 -> [g]  "<g>"
  Bus Selector/10 -> [l]  "<l>"
  Bus Selector/11 -> [Iwf]  "<Iwf>"
  Bus Selector/12 -> [Iwr]  "<Iwr>"
  wheel/1(Fl) -> body_chassis_vert/4, [Fl]
  Bus Selector1/1 -> Bus Creator2/2  "<vx>"
  Bus Selector1/2 -> Bus Creator3/2  "<vy>"
  Bus Selector1/3 -> Bus Creator4/2  "<vz>"
  Bus Selector2/1 -> Bus Creator2/3  "<ax>"
  Bus Selector2/2 -> [ay], Bus Creator3/3  "<ay>"
  Bus Selector2/3 -> Bus Creator4/3  "<az>"
  reset/1 -> [reset], To Workspace3/1
  body_chassis_vert/11 -> wheel/11(Fzt), [Fz], Bus to Vector18/1
  Überlagerung/1(ges_lenkwinkel) -> body_chassis_vert/3, delta_kinematic/1, [delta], Bus to Vector/1, wheel/3(delta)
  FZG_delta/1 -> [delta_d], Überlagerung/2(lenkwinkel)
  Bus to Vector/1 -> To Workspace11/1
  Bus to Vector1/1 -> To Workspace14/1
  Bus to Vector2/1 -> To Workspace21/1
  Bus to Vector3/1 -> To Workspace22/1
  Bus to Vector4/1 -> To Workspace31/1
  Bus to Vector6/1 -> To Workspace23/1
  Bus to Vector7/1 -> To Workspace24/1
  Bus to Vector8/1 -> To Workspace25/1
  Bus to Vector16/1 -> To Workspace26/1
  Bus to Vector17/1 -> To Workspace16/1
  Bus to Vector18/1 -> To Workspace32/1
  Bus to Vector19/1 -> To Workspace17/1
  Bus to Vector20/1 -> To Workspace15/1
  Bus to Vector21/1 -> To Workspace29/1
  Bus to Vector22/1 -> To Workspace27/1
  Bus to Vector23/1 -> To Workspace20/1
  Bus to Vector24/1 -> To Workspace19/1
  Bus to Vector25/1 -> To Workspace18/1
  Bus Selector/35 -> [sarbR]  "<sarbR>"
  wheel/16(fric_save) -> [fric_save]
  [F0] -> F0/1

== system vehicle_model/simplified_vehicle_model/Correction_subsystem ==
  P_damper : Inport
  Bus Creator1 : BusCreator  Inputs=4
  Bus Selector4 : BusSelector  OutputSignals=P_damper_Front,P_damper_Rear
  Signal Conversion{1..3,7} (4 alike) : SignalConversion  OverrideOpt=off
  P_damper_korr : Outport
  wires:
  Bus Creator1/1 -> P_damper_korr/1
  Bus Selector4/2 -> Signal Conversion1/1, Signal Conversion2/1  "<P_damper_Rear>"
  Signal Conversion7/1 -> Bus Creator1/2  "P_damper_LF"
  Signal Conversion1/1 -> Bus Creator1/4  "P_damper_LR"
  Bus Selector4/1 -> Signal Conversion7/1, Signal Conversion3/1  "<P_damper_Front>"
  P_damper/1 -> Bus Selector4/1
  Signal Conversion2/1 -> Bus Creator1/3  "P_damper_RR"
  Signal Conversion3/1 -> Bus Creator1/1  "P_damper_RF"

== system vehicle_model/simplified_vehicle_model/Correction_subsystem1 ==
  Fz : Inport
  Bus Creator1 : BusCreator  Inputs=4
  Bus Selector4 : BusSelector  OutputSignals=Fz_Front,Fz_Rear
  Signal Conversion{1..3,7} (4 alike) : SignalConversion  OverrideOpt=off
  Fz_korr : Outport
  wires:
  Bus Creator1/1 -> Fz_korr/1
  Bus Selector4/2 -> Signal Conversion1/1, Signal Conversion2/1  "<Fz_Rear>"
  Signal Conversion7/1 -> Bus Creator1/2  "Fz_LF"
  Signal Conversion1/1 -> Bus Creator1/4  "Fz_LR"
  Bus Selector4/1 -> Signal Conversion7/1, Signal Conversion3/1  "<Fz_Front>"
  Fz/1 -> Bus Selector4/1
  Signal Conversion2/1 -> Bus Creator1/3  "Fz_RR"
  Signal Conversion3/1 -> Bus Creator1/1  "Fz_RF"

== system vehicle_model/simplified_vehicle_model/Correction_subsystem10 ==
  kappa : Inport
  Bus Creator1 : BusCreator  Inputs=4
  Bus Selector4 : BusSelector  OutputSignals=kappa_F,kappa_R
  Signal Conversion{1..3,7} (4 alike) : SignalConversion  OverrideOpt=off
  kappa_korr : Outport
  wires:
  Bus Creator1/1 -> kappa_korr/1
  Bus Selector4/2 -> Signal Conversion1/1, Signal Conversion2/1  "<kappa_R>"
  Signal Conversion7/1 -> Bus Creator1/2  "kappa_LF"
  Signal Conversion1/1 -> Bus Creator1/4  "kappa_LR"
  Bus Selector4/1 -> Signal Conversion7/1, Signal Conversion3/1  "<kappa_F>"
  kappa/1 -> Bus Selector4/1
  Signal Conversion2/1 -> Bus Creator1/3  "kappa_RR"
  Signal Conversion3/1 -> Bus Creator1/1  "kappa_RF"

== system vehicle_model/simplified_vehicle_model/Correction_subsystem11 ==
  omega : Inport
  Bus Creator1 : BusCreator  Inputs=4
  Bus Selector4 : BusSelector  OutputSignals=omega_F,omega_R
  Signal Conversion{1..3,7} (4 alike) : SignalConversion  OverrideOpt=off
  omega_korr : Outport
  wires:
  Bus Creator1/1 -> omega_korr/1
  Bus Selector4/2 -> Signal Conversion1/1, Signal Conversion2/1  "<omega_R>"
  Signal Conversion7/1 -> Bus Creator1/2  "omega_LF"
  Signal Conversion1/1 -> Bus Creator1/4  "omega_LR"
  Bus Selector4/1 -> Signal Conversion7/1, Signal Conversion3/1  "<omega_F>"
  omega/1 -> Bus Selector4/1
  Signal Conversion2/1 -> Bus Creator1/3  "omega_RR"
  Signal Conversion3/1 -> Bus Creator1/1  "omega_RF"

== system vehicle_model/simplified_vehicle_model/Correction_subsystem12 ==
  r_dyn : Inport
  Bus Creator1 : BusCreator  Inputs=4
  Bus Selector4 : BusSelector  OutputSignals=r_dyn_F,r_dyn_R
  Signal Conversion{1..3,7} (4 alike) : SignalConversion  OverrideOpt=off
  r_dyn_korr : Outport
  wires:
  Bus Creator1/1 -> r_dyn_korr/1
  Bus Selector4/2 -> Signal Conversion1/1, Signal Conversion2/1  "<r_dyn_R>"
  Signal Conversion7/1 -> Bus Creator1/2  "r_dyn_LF"
  Signal Conversion1/1 -> Bus Creator1/4  "r_dyn_LR"
  Bus Selector4/1 -> Signal Conversion7/1, Signal Conversion3/1  "<r_dyn_F>"
  r_dyn/1 -> Bus Selector4/1
  Signal Conversion2/1 -> Bus Creator1/3  "r_dyn_RR"
  Signal Conversion3/1 -> Bus Creator1/1  "r_dyn_RF"

== system vehicle_model/simplified_vehicle_model/Correction_subsystem13 ==
  vl : Inport
  Bus Creator1 : BusCreator  Inputs=4
  Bus Selector4 : BusSelector  OutputSignals=vx
  Signal Conversion{1..3,7} (4 alike) : SignalConversion  OverrideOpt=off
  vl_korr : Outport
  wires:
  Bus Creator1/1 -> vl_korr/1
  Signal Conversion7/1 -> Bus Creator1/2  "vl_LF"
  Signal Conversion1/1 -> Bus Creator1/4  "vl_LR"
  Bus Selector4/1 -> Signal Conversion1/1, Signal Conversion2/1, Signal Conversion7/1, Signal Conversion3/1  "<vx>"
  vl/1 -> Bus Selector4/1
  Signal Conversion2/1 -> Bus Creator1/3  "vl_RR"
  Signal Conversion3/1 -> Bus Creator1/1  "vl_RF"

== system vehicle_model/simplified_vehicle_model/Correction_subsystem14 ==
  z_wheel : Inport
  Bus Creator1 : BusCreator  Inputs=4
  Bus Selector4 : BusSelector  OutputSignals=z_wheel_Front,z_wheel_Rear
  Signal Conversion{1..3,7} (4 alike) : SignalConversion  OverrideOpt=off
  z_wheel_korr : Outport
  wires:
  Bus Creator1/1 -> z_wheel_korr/1
  Bus Selector4/2 -> Signal Conversion1/1, Signal Conversion2/1  "<z_wheel_Rear>"
  Signal Conversion7/1 -> Bus Creator1/2  "z_wheel_LF"
  Signal Conversion1/1 -> Bus Creator1/4  "z_wheel_LR"
  Bus Selector4/1 -> Signal Conversion7/1, Signal Conversion3/1  "<z_wheel_Front>"
  z_wheel/1 -> Bus Selector4/1
  Signal Conversion2/1 -> Bus Creator1/3  "z_wheel_RR"
  Signal Conversion3/1 -> Bus Creator1/1  "z_wheel_RF"

== system vehicle_model/simplified_vehicle_model/Correction_subsystem15 ==
  gamma : Inport
  Bus Creator1 : BusCreator  Inputs=4
  Bus Selector4 : BusSelector  OutputSignals=gamma_F,gamma_R
  Gain : Gain  Gain=-1
  Gain1 : Gain  Gain=-1
  Signal Conversion{1..3,7} (4 alike) : SignalConversion  OverrideOpt=off
  gamma_korr : Outport
  wires:
  Bus Creator1/1 -> gamma_korr/1
  Bus Selector4/2 -> Gain1/1, Signal Conversion2/1  "<gamma_R>"
  Signal Conversion7/1 -> Bus Creator1/2  "gamma_LF"
  Signal Conversion1/1 -> Bus Creator1/4  "gamma_LR"
  Bus Selector4/1 -> Gain/1, Signal Conversion3/1  "<gamma_F>"
  gamma/1 -> Bus Selector4/1
  Signal Conversion2/1 -> Bus Creator1/3  "gamma_RR"
  Signal Conversion3/1 -> Bus Creator1/1  "gamma_RF"
  Gain/1 -> Signal Conversion7/1
  Gain1/1 -> Signal Conversion1/1

== system vehicle_model/simplified_vehicle_model/Correction_subsystem2 ==
  Fl : Inport
  Bus Creator1 : BusCreator  Inputs=4
  Bus Selector4 : BusSelector  OutputSignals=Fl_F,Fl_R
  Signal Conversion{1..3,7} (4 alike) : SignalConversion  OverrideOpt=off
  Fl_korr : Outport
  wires:
  Bus Creator1/1 -> Fl_korr/1
  Bus Selector4/2 -> Signal Conversion1/1, Signal Conversion2/1  "<Fl_R>"
  Signal Conversion7/1 -> Bus Creator1/2  "Fl_LF"
  Signal Conversion1/1 -> Bus Creator1/4  "Fl_LR"
  Bus Selector4/1 -> Signal Conversion7/1, Signal Conversion3/1  "<Fl_F>"
  Fl/1 -> Bus Selector4/1
  Signal Conversion2/1 -> Bus Creator1/3  "Fl_RR"
  Signal Conversion3/1 -> Bus Creator1/1  "Fl_RF"

== system vehicle_model/simplified_vehicle_model/Correction_subsystem3 ==
  Fs : Inport
  Bus Creator1 : BusCreator  Inputs=4
  Bus Selector4 : BusSelector  OutputSignals=Fs_F,Fs_R
  Gain : Gain  Gain=-1
  Gain1 : Gain  Gain=-1
  Signal Conversion{1..3,7} (4 alike) : SignalConversion  OverrideOpt=off
  Fs_korr : Outport
  wires:
  Bus Creator1/1 -> Fs_korr/1
  Bus Selector4/2 -> Gain1/1, Signal Conversion2/1  "<Fs_R>"
  Signal Conversion7/1 -> Bus Creator1/2  "Fs_LF"
  Signal Conversion1/1 -> Bus Creator1/4  "Fs_LR"
  Bus Selector4/1 -> Gain/1, Signal Conversion3/1  "<Fs_F>"
  Fs/1 -> Bus Selector4/1
  Signal Conversion2/1 -> Bus Creator1/3  "Fs_RR"
  Signal Conversion3/1 -> Bus Creator1/1  "Fs_RF"
  Gain/1 -> Signal Conversion7/1
  Gain1/1 -> Signal Conversion1/1

== system vehicle_model/simplified_vehicle_model/Correction_subsystem4 ==
  Mx : Inport
  Bus Creator1 : BusCreator  Inputs=4
  Bus Selector4 : BusSelector  OutputSignals=Ml_F,Ml_R
  Gain : Gain  Gain=-1
  Gain1 : Gain  Gain=-1
  Signal Conversion{1..3,7} (4 alike) : SignalConversion  OverrideOpt=off
  Mx_korr : Outport
  wires:
  Bus Creator1/1 -> Mx_korr/1
  Bus Selector4/2 -> Gain1/1, Signal Conversion2/1  "<Ml_R>"
  Signal Conversion7/1 -> Bus Creator1/2  "Mx_LF"
  Signal Conversion1/1 -> Bus Creator1/4  "Mx_LR"
  Bus Selector4/1 -> Signal Conversion3/1, Gain/1  "<Ml_F>"
  Mx/1 -> Bus Selector4/1
  Signal Conversion2/1 -> Bus Creator1/3  "Mx_RR"
  Signal Conversion3/1 -> Bus Creator1/1  "Mx_RF"
  Gain/1 -> Signal Conversion7/1
  Gain1/1 -> Signal Conversion1/1

== system vehicle_model/simplified_vehicle_model/Correction_subsystem5 ==
  My : Inport
  Bus Creator1 : BusCreator  Inputs=4
  Bus Selector4 : BusSelector  OutputSignals=Ms_F,Ms_R
  Signal Conversion{1..3,7} (4 alike) : SignalConversion  OverrideOpt=off
  My_korr : Outport
  wires:
  Bus Creator1/1 -> My_korr/1
  Bus Selector4/2 -> Signal Conversion1/1, Signal Conversion2/1  "<Ms_R>"
  Signal Conversion7/1 -> Bus Creator1/2  "My_LF"
  Signal Conversion1/1 -> Bus Creator1/4  "My_LR"
  Bus Selector4/1 -> Signal Conversion7/1, Signal Conversion3/1  "<Ms_F>"
  My/1 -> Bus Selector4/1
  Signal Conversion2/1 -> Bus Creator1/3  "My_RR"
  Signal Conversion3/1 -> Bus Creator1/1  "My_RF"

== system vehicle_model/simplified_vehicle_model/Correction_subsystem6 ==
  Mz : Inport
  Bus Creator1 : BusCreator  Inputs=4
  Bus Selector4 : BusSelector  OutputSignals=Mv_F,Mv_R
  Gain : Gain  Gain=-1
  Gain1 : Gain  Gain=-1
  Signal Conversion{1..3,7} (4 alike) : SignalConversion  OverrideOpt=off
  Mz_korr : Outport
  wires:
  Bus Creator1/1 -> Mz_korr/1
  Bus Selector4/2 -> Gain/1, Signal Conversion2/1  "<Mv_R>"
  Signal Conversion7/1 -> Bus Creator1/2  "Mz_LF"
  Signal Conversion1/1 -> Bus Creator1/4  "Mz_LR"
  Bus Selector4/1 -> Gain1/1, Signal Conversion3/1  "<Mv_F>"
  Mz/1 -> Bus Selector4/1
  Signal Conversion2/1 -> Bus Creator1/3  "Mz_RR"
  Signal Conversion3/1 -> Bus Creator1/1  "Mz_RF"
  Gain/1 -> Signal Conversion1/1
  Gain1/1 -> Signal Conversion7/1

== system vehicle_model/simplified_vehicle_model/Correction_subsystem7 ==
  r_stat : Inport
  Bus Creator1 : BusCreator  Inputs=4
  Bus Selector4 : BusSelector  OutputSignals=r_stat_F,r_stat_R
  Signal Conversion{1..3,7} (4 alike) : SignalConversion  OverrideOpt=off
  r_stat_korr : Outport
  wires:
  Bus Creator1/1 -> r_stat_korr/1
  Bus Selector4/2 -> Signal Conversion1/1, Signal Conversion2/1  "<r_stat_R>"
  Signal Conversion7/1 -> Bus Creator1/2  "r_stat_LF"
  Signal Conversion1/1 -> Bus Creator1/4  "r_stat_LR"
  Bus Selector4/1 -> Signal Conversion7/1, Signal Conversion3/1  "<r_stat_F>"
  r_stat/1 -> Bus Selector4/1
  Signal Conversion2/1 -> Bus Creator1/3  "r_stat_RR"
  Signal Conversion3/1 -> Bus Creator1/1  "r_stat_RF"

== system vehicle_model/simplified_vehicle_model/Correction_subsystem8 ==
  F0 : Inport
  Bus Creator1 : BusCreator  Inputs=4
  Bus Selector4 : BusSelector  OutputSignals=F,R
  Signal Conversion{1..3,7} (4 alike) : SignalConversion  OverrideOpt=off
  F0_korr : Outport
  wires:
  Bus Creator1/1 -> F0_korr/1
  Bus Selector4/2 -> Signal Conversion1/1, Signal Conversion2/1  "<R>"
  Signal Conversion7/1 -> Bus Creator1/2  "LF"
  Signal Conversion1/1 -> Bus Creator1/4  "LR"
  Bus Selector4/1 -> Signal Conversion7/1, Signal Conversion3/1  "<F>"
  F0/1 -> Bus Selector4/1
  Signal Conversion2/1 -> Bus Creator1/3  "RR"
  Signal Conversion3/1 -> Bus Creator1/1  "RF"

== system vehicle_model/simplified_vehicle_model/Correction_subsystem9 ==
  alpha : Inport
  Bus Creator1 : BusCreator  Inputs=4
  Bus Selector4 : BusSelector  OutputSignals=alpha_F,alpha_R
  Signal Conversion{1..3,7} (4 alike) : SignalConversion  OverrideOpt=off
  alpha_korr : Outport
  wires:
  Bus Creator1/1 -> alpha_korr/1
  Bus Selector4/2 -> Signal Conversion1/1, Signal Conversion2/1  "<alpha_R>"
  Signal Conversion7/1 -> Bus Creator1/2  "alpha_LF"
  Signal Conversion1/1 -> Bus Creator1/4  "alpha_LR"
  Bus Selector4/1 -> Signal Conversion7/1, Signal Conversion3/1  "<alpha_F>"
  alpha/1 -> Bus Selector4/1
  Signal Conversion2/1 -> Bus Creator1/3  "alpha_RR"
  Signal Conversion3/1 -> Bus Creator1/1  "alpha_RF"
